simulink model "desulfuradora"  (Simulink 8.5)
settings: Solver=ode45  StartTime=0.0  StopTime=20000  RelTol=1e-3
undefined symbols (not defined in the file or in its folder): magnitude, Pump, SmartFuel, tabla, tank
settings Model: Creator=juanillo  LastModifiedBy=Jota
settings OptimizationCC: InitFltsAndDblsToZero=on
settings DebuggingCC: SaveWithParameterizedLinksMsg=none  SolverPrmCheckMsg=warning  FcnCallInpInsideContextMsg=UseLocalSettings
settings GRTTargetCC: TargetFcnLib=ansi_tfl_tmw.mat

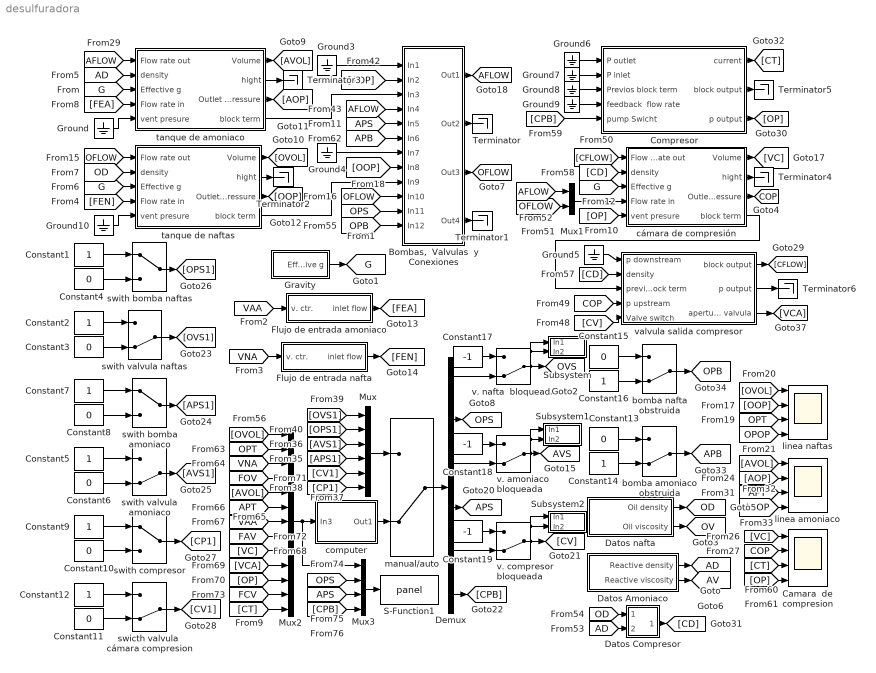
== system desulfuradora ==
  " bomba amoniaco obstruida" : ManualSwitch  CurrentSetting=0
  " bomba nafta obstruida" : ManualSwitch  CurrentSetting=0
  " linea amoniaco" : Scope  NumInputPorts=4
      settings: TickLabels=on  YMin=19~93100~36.9~210808  YMax=21~102900~37.1~232998  SaveName=tnafta2
  " linea naftas" : Scope  NumInputPorts=4
      settings: TickLabels=on  YMin=1~0~20~0  YMax=11~55000~110~200000  SaveName=tnafta
  " v. amoniaco  bloqueada" : ManualSwitch  CurrentSetting=0
  " v. compresor  bloqueada" : ManualSwitch  CurrentSetting=0
  " v. nafta  bloqueada" : ManualSwitch  CurrentSetting=0
  "Bombas,  Valvulas  y Conexiones" : Subsystem
  Camara  de compresion : Scope  NumInputPorts=4
      settings: TimeRange=2000  YMin=17.1501~1.45e+007~145~1.45e+007  YMax=18.9553~2.05e+007~162.5~2.05e+007  SaveName=camarac
  Compresor : Subsystem  AncestorBlock=SmartFuel/Pump  mask{V=350, P=2000, Rc=2, RO=0.2, L=20, Kb=0.35, Ki=0.5, J=2.5, A=2, R=250, E=0}
      mask prompts: V "Nominal Voltage"; P "Nominal Power"; Rc "rotor elec resistance"; RO "rotor mec. resitance"; L "rotor inductance"; Kb "Ind constant"; Ki "magres"; J "Rotor inertia"; A "valve section"; R "pump efficiency"; E "Last element (0/1)"
  Constant{1..2,5,7,9,12,14,16} (8 alike) : Constant
  Constant{3..4,6,8,10..11,13,15} (8 alike) : Constant  Value=0
  Constant17 : Constant  Value=-1
  Constant18 : Constant  Value=-1
  Constant19 : Constant  Value=-1
  Datos Amoniaco : Subsystem  AncestorBlock=SmartFuel/Fuel data  mask{ro=1000, mu=1.3}
      mask prompts: ro "Fuel density"; mu "Fuel viscosity"
  Datos Compresor : Subsystem
  Datos nafta : Subsystem  AncestorBlock=SmartFuel/Fuel data  mask{ro=1000, mu=1.3}
      mask prompts: ro "Fuel density"; mu "Fuel viscosity"
  Demux : Demux  Outputs=6
  Flujo de entrada amoniaco : Subsystem  mask{T=40, C=0.6}
      mask prompts: T "Inlet Period"; C "Flow"
  Flujo de entrada nafta : Subsystem  mask{T=40, C=0.4}
      mask prompts: T "Inlet period"; C "Flow"
  Gravity : Subsystem  AncestorBlock=SmartFuel/Aircraft data  mask{g=9.8, atitude=[0 0 0]}
      mask prompts: g "effective g"; atitude "Aircraft atitude"
  Ground{,3..10} (9 alike) : Ground
  Mux : Mux  Inputs=6
  Mux1 : Mux  Inputs=2
  Mux2 : Mux  Inputs=13
  Mux3 : Mux
  S-Function1 : S-Function  FunctionName=panel
  Subsystem : Subsystem
      mask Display: disp('FOV')
  Subsystem1 : Subsystem
      mask Display: disp('FAV')
  Subsystem2 : Subsystem
      mask Display: disp('FCV')
  Terminator{,1..6} (7 alike) : Terminator
  computer : Subsystem
      mask Display: disp('ordenador\n de control')
  cámara de compresión : Subsystem  AncestorBlock=SmartFuel/tank  mask{S=2, max=20, V0=0}
      mask prompts: S "Tank Geometrical Parameters"; max "Tank Max. Volume"; V0 "Initial Vol."
  manual/auto : ManualSwitch  CurrentSetting=0
  "swicth valvula  cámara compresion " : ManualSwitch  CurrentSetting=0
  swith bomba amoniaco : ManualSwitch
  swith bomba naftas : ManualSwitch
  swith compresor : ManualSwitch
  swith valvula amoniaco : ManualSwitch  CurrentSetting=0
  swith valvula naftas : ManualSwitch  CurrentSetting=0
  tanque de amoniaco : Subsystem  AncestorBlock=SmartFuel/tank  mask{S=2, max=20, V0=1}
      mask prompts: S "Tank Geometrical Parameters"; max "Tank Max. Volume"; V0 "Initial Vol."
  tanque de naftas : Subsystem  AncestorBlock=SmartFuel/tank  mask{S=2, max=20, V0=1}
      mask prompts: S "Tank Geometrical Parameters"; max "Tank Max. Volume"; V0 "Initial Vol."
  valvula salida compresor : Subsystem  mask{cv=0.5, T=0.1, A=0.2, E=1}
      mask prompts: cv "valve resistence"; T "aperture time"; A "Maximum valve aperture"; E "Last block (0/1)"
  tag scope: AD=global, AFLOW=global, APB=global, APS=global, AV=global, AVS=global, COP=global, G=global, OD=global, OFLOW=global, OPB=global, OPS=global, OV=global, OVS=global
  wires:
  Datos Amoniaco/1(Reactive density) -> [AD]
  Gravity/1(Effective g) -> [G]
  Datos Amoniaco/2(Reactive viscosity) -> [AV]
  Datos nafta/1(Oil density) -> [OD]
  Datos nafta/2(Oil viscosity) -> [OV]
  [AD] -> tanque de amoniaco/2(" density")
  [G] -> tanque de amoniaco/3(Effective g)
  [OD] -> tanque de naftas/2(" density")
  [G] -> tanque de naftas/3(Effective g)
  tanque de naftas/4(block term) -> "Bombas,  Valvulas  y Conexiones"/9(In9)
  cámara de compresión/3(Outlet Pressure) -> [COP]
  Mux1/1 -> cámara de compresión/4(Flow rate in)
  [G] -> cámara de compresión/3(Effective g)
  [OFLOW] -> tanque de naftas/1(Flow rate out)
  swith valvula naftas/1 -> [OVS1]
  Constant2/1 -> swith valvula naftas/1
  Constant3/1 -> swith valvula naftas/2
  cámara de compresión/1(Volume) -> [VC]
  tanque de amoniaco/1(Volume) -> [AVOL]
  tanque de naftas/1(Volume) -> [OVOL]
  tanque de amoniaco/3(Outlet Pressure) -> [AOP]
  tanque de naftas/3(Outlet Pressure) -> [OOP]
  [OPT] -> " linea naftas"/3
  [VC] -> Camara  de compresion/1
  [COP] -> Camara  de compresion/2
  [AFLOW] -> tanque de amoniaco/1(Flow rate out)
  [OVOL] -> " linea naftas"/1
  [OOP] -> " linea naftas"/2
  swith bomba naftas/1 -> [OPS1]
  Constant1/1 -> swith bomba naftas/1
  Constant4/1 -> swith bomba naftas/2
  swith valvula amoniaco/1 -> [AVS1]
  Constant5/1 -> swith valvula amoniaco/1
  Constant6/1 -> swith valvula amoniaco/2
  [APT] -> " linea amoniaco"/3
  [AVOL] -> " linea amoniaco"/1
  [AOP] -> " linea amoniaco"/2
  [APOP] -> " linea amoniaco"/4
  swith bomba amoniaco/1 -> [APS1]
  Constant7/1 -> swith bomba amoniaco/1
  Constant8/1 -> swith bomba amoniaco/2
  swith compresor/1 -> [CP1]
  Constant9/1 -> swith compresor/1
  Constant10/1 -> swith compresor/2
  Ground/1 -> tanque de amoniaco/5(vent presure)
  tanque de amoniaco/4(block term) -> "Bombas,  Valvulas  y Conexiones"/3(In3)
  Mux/1 -> manual/auto/1
  Demux/2 -> [OPS]
  Demux/3 -> " v. amoniaco  bloqueada"/2
  Demux/4 -> [APS]
  "swicth valvula  cámara compresion "/1 -> [CV1]
  Constant12/1 -> "swicth valvula  cámara compresion "/1
  Constant11/1 -> "swicth valvula  cámara compresion "/2
  Demux/6 -> [CPB]
  [OVS1] -> Mux/1
  [OPS1] -> Mux/2
  [AVS1] -> Mux/3
  [CV1] -> Mux/5
  [CP1] -> Mux/6
  [APS1] -> Mux/4
  tanque de naftas/2(hight) -> Terminator2/1
  tanque de amoniaco/2(hight) -> Terminator3/1
  valvula salida compresor/1(block output) -> [CFLOW]
  [CV] -> valvula salida compresor/5(Valve switch)
  Ground5/1 -> valvula salida compresor/1(p downstream)
  [COP] -> valvula salida compresor/4(p upstream)
  cámara de compresión/4(block term) -> valvula salida compresor/3(previous block term)
  cámara de compresión/2(hight) -> Terminator4/1
  Compresor/2(block output) -> Terminator5/1
  Compresor/3(p output) -> [OP]
  [OP] -> cámara de compresión/5(vent presure)
  [CFLOW] -> cámara de compresión/1(Flow rate out)
  [OFLOW] -> Mux1/2
  [AFLOW] -> Mux1/1
  Datos Compresor/1(Out3) -> [CD]
  [CD] -> cámara de compresión/2(" density")
  [CD] -> valvula salida compresor/2(" density")
  Ground6/1 -> Compresor/1(P outlet)
  Ground7/1 -> Compresor/2(P inlet)
  Ground8/1 -> Compresor/3(Previos block term)
  Ground9/1 -> Compresor/4(feedback  flow rate)
  [CPB] -> Compresor/5(pump Swicht)
  Compresor/1(current) -> [CT]
  [CT] -> Camara  de compresion/3
  [OP] -> Camara  de compresion/4
  Ground10/1 -> tanque de naftas/5(vent presure)
  " bomba amoniaco obstruida"/1 -> [APB]
  Constant13/1 -> " bomba amoniaco obstruida"/1
  Constant14/1 -> " bomba amoniaco obstruida"/2
  [AD] -> Datos Compresor/2(In2)
  [OD] -> Datos Compresor/1(In1)
  " bomba nafta obstruida"/1 -> [OPB]
  Constant15/1 -> " bomba nafta obstruida"/1
  Constant16/1 -> " bomba nafta obstruida"/2
  Mux2/1 -> Mux3/1, computer/1(In3)
  computer/1(Out1) -> manual/auto/2
  [OVOL] -> Mux2/1
  [OPT] -> Mux2/2
  " v. nafta  bloqueada"/1 -> Subsystem/2(In2), Subsystem/1(In1), [OVS]
  Demux/1 -> " v. nafta  bloqueada"/2
  Constant17/1 -> " v. nafta  bloqueada"/1
  " v. amoniaco  bloqueada"/1 -> [AVS], Subsystem1/2(In2), Subsystem1/1(In1)
  Constant18/1 -> " v. amoniaco  bloqueada"/1
  Demux/5 -> " v. compresor  bloqueada"/2
  " v. compresor  bloqueada"/1 -> [CV], Subsystem2/2(In2), Subsystem2/1(In1)
  [VNA] -> Mux2/3
  valvula salida compresor/3(apertura valvula) -> [VCA]
  valvula salida compresor/2(p output) -> Terminator6/1
  [AVOL] -> Mux2/5
  [APT] -> Mux2/6
  [VAA] -> Mux2/7
  [FOV] -> Mux2/4
  [VC] -> Mux2/9
  [VCA] -> Mux2/10
  [OP] -> Mux2/11
  [FAV] -> Mux2/8
  [FCV] -> Mux2/12
  [OPOP] -> " linea naftas"/4
  Mux3/1 -> S-Function1/1
  [OPS] -> Mux3/2
  [APS] -> Mux3/3
  [CPB] -> Mux3/4
  Constant19/1 -> " v. compresor  bloqueada"/1
  [APB] -> "Bombas,  Valvulas  y Conexiones"/6(In6)
  "Bombas,  Valvulas  y Conexiones"/2(Out2) -> Terminator/1
  Ground3/1 -> "Bombas,  Valvulas  y Conexiones"/1(In1)
  [AFLOW] -> "Bombas,  Valvulas  y Conexiones"/4(In4)
  [AOP] -> "Bombas,  Valvulas  y Conexiones"/2(In2)
  [APS] -> "Bombas,  Valvulas  y Conexiones"/5(In5)
  "Bombas,  Valvulas  y Conexiones"/1(Out1) -> [AFLOW]
  [OPB] -> "Bombas,  Valvulas  y Conexiones"/12(In12)
  "Bombas,  Valvulas  y Conexiones"/4(Out4) -> Terminator1/1
  Ground4/1 -> "Bombas,  Valvulas  y Conexiones"/7(In7)
  [OOP] -> "Bombas,  Valvulas  y Conexiones"/8(In8)
  [OFLOW] -> "Bombas,  Valvulas  y Conexiones"/10(In10)
  "Bombas,  Valvulas  y Conexiones"/3(Out3) -> [OFLOW]
  [OPS] -> "Bombas,  Valvulas  y Conexiones"/11(In11)
  manual/auto/1 -> Demux/1
  [VAA] -> Flujo de entrada amoniaco/1(v. ctr.)
  [VNA] -> Flujo de entrada nafta/1(v. ctr.)
  Flujo de entrada amoniaco/1(inlet flow) -> [FEA]
  Flujo de entrada nafta/1(inlet flow) -> [FEN]
  [FEN] -> tanque de naftas/4(Flow rate in)
  [FEA] -> tanque de amoniaco/4(Flow rate in)
  [CT] -> Mux2/13

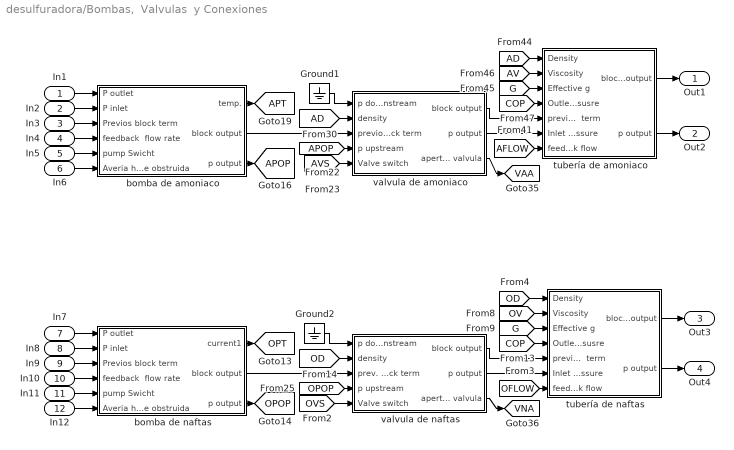
== system desulfuradora/Bombas,  Valvulas  y Conexiones ==
  In1 : Inport
  In2 : Inport  Port=2
  In3 : Inport  Port=3
  In4 : Inport  Port=4
  In5 : Inport  Port=5
  In6 : Inport  Port=6
  In7 : Inport  Port=7
  In8 : Inport  Port=8
  In9 : Inport  Port=9
  In10 : Inport  Port=10
  In11 : Inport  Port=11
  In12 : Inport  Port=12
  Ground1 : Ground
  Ground2 : Ground
  bomba de amoniaco : Subsystem  AncestorBlock=SmartFuel/Pump  mask{V=250, P=5000, Rc=2, RO=0.2, L=2, Kb=0.5, Ki=8, J=2.5, A=0.3, R=0.6, E=0}
      mask prompts: V "Nominal Voltage"; P "Nominal Power"; Rc "rotor elec resistance"; RO "rotor mec. resitance"; L "rotor inductance"; Kb "Ind constant"; Ki "magres"; J "Rotor inertia"; A "valve section"; R "pump efficiency"; E "Last element (0/1)"
  bomba de naftas : Subsystem  AncestorBlock=SmartFuel/Pump  mask{V=250, P=5000, Rc=2, RO=0.2, L=2, Kb=0.5, Ki=8, J=2.5, A=0.3, R=0.6, E=0}
      mask prompts: V "Nominal Voltage"; P "Nominal Power"; Rc "rotor elec resistance"; RO "rotor mec. resitance"; L "rotor inductance"; Kb "Ind constant"; Ki "magres"; J "Rotor inertia"; A "valve section"; R "pump efficiency"; E "Last element (0/1)"
  tubería de amoniaco : Subsystem  mask{PA=[0  0  0], D=0.3, L=2, R=0.00003, E=1}
      mask prompts: PA "Pipe atitude (Relative to landed aircraft)"; D "Pipe Diameter"; L "Pipe Length"; R "Pipe Rougness"; E "Last block (0/1)"
      mask init:
      | load re
      | load tabla
      | load eps_d
  tubería de naftas : Subsystem  mask{PA=[0  0  0], D=0.3, L=2, R=0.00003, E=1}
      mask prompts: PA "Pipe atitude (Relative to landed aircraft)"; D "Pipe Diameter"; L "Pipe Length"; R "Pipe Rougness"; E "Last block (0/1)"
      mask init:
      | load re
      | load tabla
      | load eps_d
  valvula de amoniaco : Subsystem  mask{cv=0.5, T=0.1, A=0.3, E=0}
      mask prompts: cv "valve resistence"; T "aperture time"; A "Maximum valve aperture"; E "Last block (0/1)"
  valvula de naftas : Subsystem  mask{cv=0.5, T=0.1, A=0.3, E=0}
      mask prompts: cv "valve resistence"; T "aperture time"; A "Maximum valve aperture"; E "Last block (0/1)"
  Out1 : Outport
  Out2 : Outport  Port=2
  Out3 : Outport  Port=3
  Out4 : Outport  Port=4
  tag scope: APOP=global, APT=global, OPOP=global, OPT=global, VAA=global, VNA=global
  wires:
  [AD] -> tubería de amoniaco/1(Density)
  valvula de amoniaco/3(apertura valvula) -> [VAA]
  valvula de amoniaco/1(block output) -> tubería de amoniaco/5(previous block  term)
  [COP] -> tubería de amoniaco/4(Outlet Presusre)
  [G] -> tubería de amoniaco/3(Effective g)
  [AV] -> tubería de amoniaco/2(Viscosity)
  [AFLOW] -> tubería de amoniaco/7(feedbak flow)
  valvula de amoniaco/2(p output) -> tubería de amoniaco/6(Inlet Pressure)
  Ground1/1 -> valvula de amoniaco/1(p downstream)
  [AVS] -> valvula de amoniaco/5(Valve switch)
  [APOP] -> valvula de amoniaco/4(p upstream)
  [AD] -> valvula de amoniaco/2(" density")
  bomba de amoniaco/2(block output) -> valvula de amoniaco/3(previous block term)
  bomba de amoniaco/3(p output) -> [APOP]
  bomba de amoniaco/1(temp.) -> [APT]
  [OD] -> tubería de naftas/1(Density)
  valvula de naftas/3(apertura valvula) -> [VNA]
  Ground2/1 -> valvula de naftas/1(p downstream)
  [OPOP] -> valvula de naftas/4(p upstream)
  bomba de naftas/3(p output) -> [OPOP]
  bomba de naftas/1(current1) -> [OPT]
  [OD] -> valvula de naftas/2(" density")
  [COP] -> tubería de naftas/4(Outlet Presusre)
  [OFLOW] -> tubería de naftas/7(feedbak flow)
  [G] -> tubería de naftas/3(Effective g)
  [OV] -> tubería de naftas/2(Viscosity)
  valvula de naftas/1(block output) -> tubería de naftas/5(previous block  term)
  valvula de naftas/2(p output) -> tubería de naftas/6(Inlet Pressure)
  bomba de naftas/2(block output) -> valvula de naftas/3(prev. block term)
  [OVS] -> valvula de naftas/5(Valve switch)
  tubería de amoniaco/1(block output) -> Out1/1
  In1/1 -> bomba de amoniaco/1(P outlet)
  In2/1 -> bomba de amoniaco/2(P inlet)
  In3/1 -> bomba de amoniaco/3(Previos block term)
  tubería de amoniaco/2(p output) -> Out2/1
  In4/1 -> bomba de amoniaco/4(feedback  flow rate)
  In5/1 -> bomba de amoniaco/5(pump Swicht)
  In6/1 -> bomba de amoniaco/6(Averia helice obstruida)
  tubería de naftas/1(block output) -> Out3/1
  In7/1 -> bomba de naftas/1(P outlet)
  In8/1 -> bomba de naftas/2(P inlet)
  In9/1 -> bomba de naftas/3(Previos block term)
  tubería de naftas/2(p output) -> Out4/1
  In10/1 -> bomba de naftas/4(feedback  flow rate)
  In11/1 -> bomba de naftas/5(pump Swicht)
  In12/1 -> bomba de naftas/6(Averia helice obstruida)

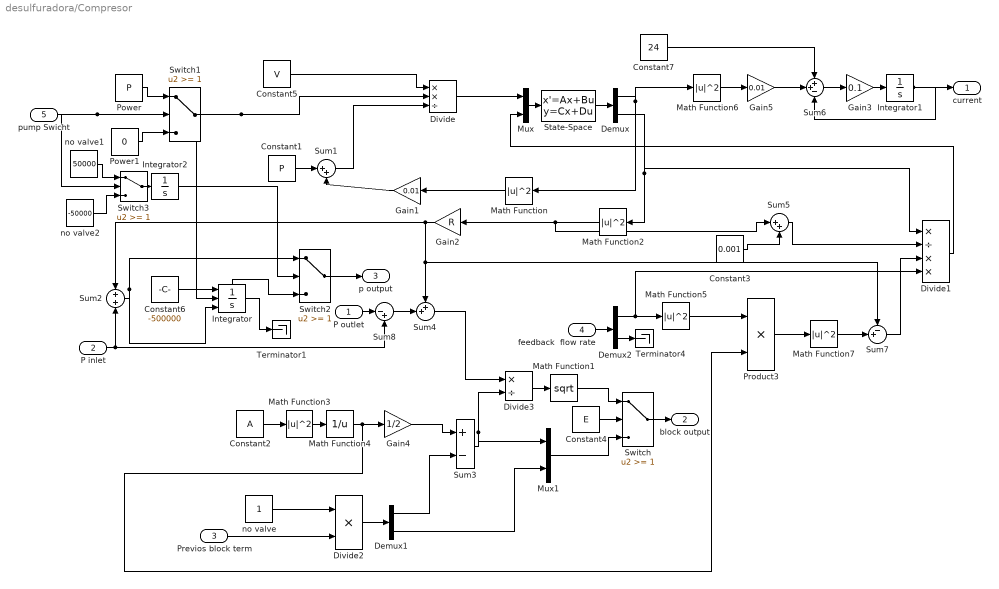
== system desulfuradora/Compresor ==
  P outlet : Inport
  P inlet : Inport  Port=2
  Previos block term : Inport  Port=3
  feedback  flow rate : Inport  Port=4
  pump Swicht : Inport  Port=5
  Constant1 : Constant  Value=P
  Constant2 : Constant  Value=A
  Constant3 : Constant  Value=0.001
  Constant4 : Constant  Value=E
  Constant5 : Constant  Value=V
  Constant6 : Constant  Value=-500000
  Constant7 : Constant  Value=24
  Demux : Demux  Outputs=2
  Demux1 : Demux  Outputs=2
  Demux2 : Demux  Outputs=2
  Divide : Product  Inputs=**/
  Divide1 : Product  Inputs=*/**
  Divide2 : Product  Inputs=**
  Divide3 : Product  Inputs=*/
  Gain1 : Gain  Gain=0.01
  Gain2 : Gain  Gain=R
  Gain3 : Gain  Gain=0.1
  Gain4 : Gain  Gain=1/2
  Gain5 : Gain  Gain=0.01
  Integrator : Integrator  ExternalReset=falling  InitialConditionSource=external  LimitOutput=on  LowerSaturationLimit=0  ShowStatePort=on
  Integrator1 : Integrator  InitialCondition=24
  Integrator2 : Integrator  LimitOutput=on  UpperSaturationLimit=1  LowerSaturationLimit=0
  Math Function{,2..3,5..7} (6 alike) : Math  Operator=magnitude^2  SaturateOnIntegerOverflow=on
  Math Function1 : Math  Operator=sqrt  SaturateOnIntegerOverflow=on
  Math Function4 : Math  Operator=reciprocal  SaturateOnIntegerOverflow=on
  Mux : Mux  Inputs=2
  Mux1 : Mux  Inputs=2
  Power : Constant  Value=P
  Power1 : Constant  Value=0
  Product3 : Product  RndMeth=Zero
  State-Space : StateSpace  A=[-Rc/L -Kb/L;Ki/J -RO/J]  B=[1/L 0;0 -1/J]  C=[1 0;0 1]  D=[0 0;0 0]  X0=0
  Sum1 : Sum  Inputs=|++
  Sum2 : Sum
  Sum3 : Sum  Inputs=+-
  Sum4 : Sum  Inputs=++|
  Sum5 : Sum  Inputs=|++
  Sum6 : Sum  Inputs=++-
  Sum7 : Sum  Inputs=-+|
  Sum8 : Sum  Inputs=|-+
  Switch{,1..3} (4 alike) : Switch  Threshold=1
  Terminator1 : Terminator
  Terminator4 : Terminator
  no valve : Constant
  no valve1 : Constant  Value=50000
  no valve2 : Constant  Value=-50000
  current : Outport
  block output : Outport  Port=2
  p output : Outport  Port=3
  wires:
  Mux/1 -> State-Space/1
  P outlet/1 -> Sum8/1
  State-Space/1 -> Demux/1
  Demux/1 -> Math Function/1, Math Function6/1
  Constant1/1 -> Sum1/1
  Demux/2 -> Divide1/1, Math Function2/1
  Math Function2/1 -> Gain2/1, Sum5/1
  P inlet/1 -> Sum2/2, Sum8/2
  Math Function3/1 -> Math Function4/1
  Math Function4/1 -> Gain4/1, Product3/2
  Constant2/1 -> Math Function3/1
  Divide2/1 -> Demux1/1
  no valve/1 -> Divide2/1
  Previos block term/1 -> Divide2/2
  Sum2/1 -> Switch2/1, Integrator/3
  Divide3/1 -> Math Function1/1
  Gain4/1 -> Sum3/1
  Sum3/1 -> Divide3/2, Mux1/1
  Constant4/1 -> Switch/2
  Switch/1 -> block output/1
  Mux1/1 -> Switch/3
  Math Function1/1 -> Switch/1
  Demux1/2 -> Mux1/2
  Power/1 -> Switch1/1
  Power1/1 -> Switch1/3
  pump Swicht/1 -> Switch1/2, Switch3/2
  feedback  flow rate/1 -> Demux2/1
  Demux2/2 -> Terminator4/1
  Demux1/1 -> Sum3/2
  Sum8/1 -> Sum4/2
  Sum4/1 -> Divide3/1
  Gain2/1 -> Sum2/1, Sum4/1, Sum7/1
  Demux2/1 -> Math Function5/1, Divide1/4
  Sum1/1 -> Divide/3
  Switch1/1 -> Divide/2, Integrator/2
  Constant5/1 -> Divide/1
  Gain1/1 -> Sum1/2
  Math Function/1 -> Gain1/1
  Divide/1 -> Mux/1
  Math Function5/1 -> Product3/1
  Product3/1 -> Math Function7/1
  Constant3/1 -> Sum5/2
  Math Function7/1 -> Sum7/2
  Sum7/1 -> Divide1/3
  Sum5/1 -> Divide1/2
  Divide1/1 -> Mux/2
  Constant6/1 -> Integrator/1
  Switch2/1 -> p output/1
  Integrator1/1 -> Sum6/3, current/1
  Constant7/1 -> Sum6/1
  Sum6/1 -> Gain3/1
  Gain3/1 -> Integrator1/1
  Gain5/1 -> Sum6/2
  Math Function6/1 -> Gain5/1
  Integrator/State -> Switch2/3
  Integrator/1 -> Terminator1/1
  Switch3/1 -> Integrator2/1
  no valve1/1 -> Switch3/1
  no valve2/1 -> Switch3/3
  Integrator2/1 -> Switch2/2

== system desulfuradora/Datos Amoniaco ==
  FD : Constant  Value=ro
  FV : Constant  Value=mu
  Reactive density : Outport
  Reactive viscosity : Outport  Port=2
  wires:
  FV/1 -> Reactive viscosity/1
  FD/1 -> Reactive density/1

== system desulfuradora/Datos Compresor ==
  In1 : Inport
  In2 : Inport  Port=2
  Gain3 : Gain  Gain=1/2
  Sum1 : Sum
  Out3 : Outport
  wires:
  In2/1 -> Sum1/2
  In1/1 -> Sum1/1
  Gain3/1 -> Out3/1
  Sum1/1 -> Gain3/1

== system desulfuradora/Datos nafta ==
  FD : Constant  Value=ro
  FV : Constant  Value=mu
  Oil density : Outport
  Oil viscosity : Outport  Port=2
  wires:
  FV/1 -> Oil viscosity/1
  FD/1 -> Oil density/1

== system desulfuradora/Flujo de entrada amoniaco ==
  v. ctr. : Inport
  Constant20 : Constant  Value=0
  Pulse Generator : DiscretePulseGenerator  PulseType=Time based  Amplitude=C  Period=T  PulseWidth=50
  Switch : Switch  Criteria=u2 > Threshold  Threshold=-1
  inlet flow : Outport
  wires:
  Pulse Generator/1 -> Switch/3
  Constant20/1 -> Switch/1
  v. ctr./1 -> Switch/2
  Switch/1 -> inlet flow/1

== system desulfuradora/Flujo de entrada nafta ==
  v. ctr. : Inport
  Constant20 : Constant  Value=0
  Pulse Generator : DiscretePulseGenerator  PulseType=Time based  Amplitude=C  Period=T  PulseWidth=50
  Switch : Switch  Criteria=u2 > Threshold  Threshold=-1
  inlet flow : Outport
  wires:
  Pulse Generator/1 -> Switch/3
  Constant20/1 -> Switch/1
  v. ctr./1 -> Switch/2
  Switch/1 -> inlet flow/1

== system desulfuradora/Gravity ==
  EG : Constant  Value=g
  Effective g : Outport
  wires:
  EG/1 -> Effective g/1

== system desulfuradora/Subsystem ==
  In1 : Inport
  In2 : Inport  Port=2
  Constant20 : Constant
  Integrator : Integrator  LimitOutput=on  UpperSaturationLimit=1  LowerSaturationLimit=-1
  Switch : Switch
  tag scope: FOV=global
  wires:
  Switch/1 -> Integrator/1
  Constant20/1 -> Switch/1
  Integrator/1 -> [FOV]
  In1/1 -> Switch/2
  In2/1 -> Switch/3

== system desulfuradora/Subsystem1 ==
  In1 : Inport
  In2 : Inport  Port=2
  Constant20 : Constant
  Integrator : Integrator  LimitOutput=on  UpperSaturationLimit=1  LowerSaturationLimit=-1
  Switch : Switch
  tag scope: FAV=global
  wires:
  Switch/1 -> Integrator/1
  Constant20/1 -> Switch/1
  Integrator/1 -> [FAV]
  In1/1 -> Switch/2
  In2/1 -> Switch/3

== system desulfuradora/Subsystem2 ==
  In1 : Inport
  In2 : Inport  Port=2
  Constant20 : Constant
  Integrator : Integrator  LimitOutput=on  UpperSaturationLimit=1  LowerSaturationLimit=-1
  Switch : Switch
  tag scope: FCV=global
  wires:
  Switch/1 -> Integrator/1
  Constant20/1 -> Switch/1
  Integrator/1 -> [FCV]
  In1/1 -> Switch/2
  In2/1 -> Switch/3

== system desulfuradora/computer ==
  In3 : Inport
  Data Store Memory : DataStoreMemory  InitialValue=[-1, -1, -1, -1, -1, -1, -1, -1, -1, -1, -1, -1]
  Data Store Read : DataStoreRead  SampleTime=0
  Data Store Write : DataStoreWrite
  Demux : Demux  Outputs=2
  Mux : Mux  Inputs=2
  S-Function : S-Function  FunctionName=controlador
  Out1 : Outport
  wires:
  S-Function/1 -> Demux/1
  Demux/2 -> Data Store Write/1
  Demux/1 -> Out1/1
  Mux/1 -> S-Function/1
  In3/1 -> Mux/1
  Data Store Read/1 -> Mux/2

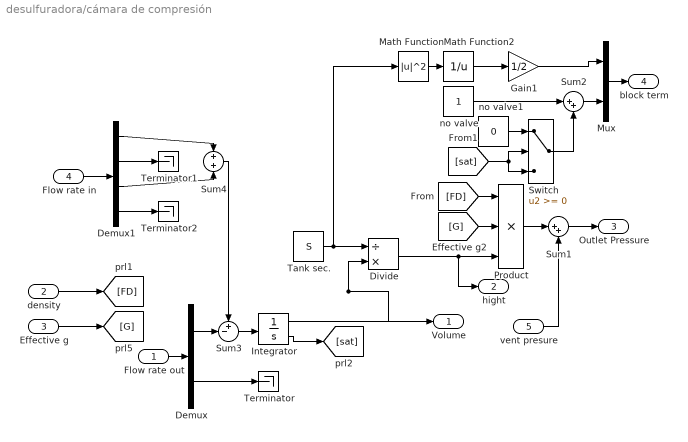
== system desulfuradora/cámara de compresión ==
  Flow rate out : Inport
  " density" : Inport  Port=2
  Effective g : Inport  Port=3
  Flow rate in : Inport  Port=4
  vent presure : Inport  Port=5
  Demux : Demux  Outputs=2
  Demux1 : Demux
  Divide : Product  Inputs=/*
  Gain1 : Gain  Gain=1/2
  Integrator : Integrator  InitialCondition=V0  LimitOutput=on  UpperSaturationLimit=max  LowerSaturationLimit=0  ShowSaturationPort=on
  Math Function1 : Math  Operator=magnitude^2  SaturateOnIntegerOverflow=on
  Math Function2 : Math  Operator=reciprocal  SaturateOnIntegerOverflow=on
  Mux : Mux  Inputs=2
  Product : Product  Inputs=3  RndMeth=Zero
  Sum1 : Sum  Inputs=|++
  Sum2 : Sum  Inputs=|++
  Sum3 : Sum  Inputs=+-|
  Sum4 : Sum
  Switch : Switch
  Tank sec. : Constant  Value=S
  Terminator : Terminator
  Terminator1 : Terminator
  Terminator2 : Terminator
  no valve : Constant
  no valve1 : Constant  Value=0
  Volume : Outport
  hight : Outport  Port=2
  Outlet Pressure : Outport  Port=3
  block term : Outport  Port=4
  wires:
  vent presure/1 -> Sum1/2
  Product/1 -> Sum1/1
  Sum1/1 -> Outlet Pressure/1
  Gain1/1 -> Mux/1
  Mux/1 -> block term/1
  Math Function2/1 -> Gain1/1
  Math Function1/1 -> Math Function2/1
  Tank sec./1 -> Math Function1/1, Divide/1
  [G] -> Product/2
  [FD] -> Product/1
  Effective g/1 -> [G]
  " density"/1 -> [FD]
  Divide/1 -> Product/3, hight/1
  Sum2/1 -> Mux/2
  no valve/1 -> Sum2/1
  Integrator/2 -> [sat]
  [sat] -> Switch/2, Switch/3
  no valve1/1 -> Switch/1
  Switch/1 -> Sum2/2
  Flow rate out/1 -> Demux/1
  Demux/2 -> Terminator/1
  Integrator/1 -> Divide/2, Volume/1
  Demux/1 -> Sum3/2
  Sum3/1 -> Integrator/1
  Flow rate in/1 -> Demux1/1
  Demux1/2 -> Terminator1/1
  Demux1/4 -> Terminator2/1
  Demux1/1 -> Sum4/1
  Demux1/3 -> Sum4/2
  Sum4/1 -> Sum3/1

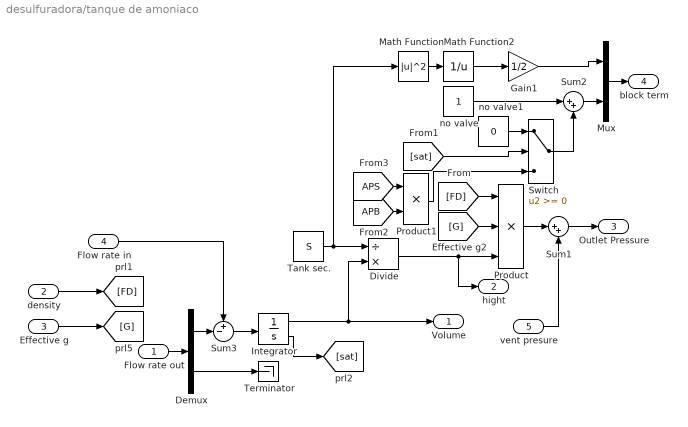
== system desulfuradora/tanque de amoniaco ==
  Flow rate out : Inport
  " density" : Inport  Port=2
  Effective g : Inport  Port=3
  Flow rate in : Inport  Port=4
  vent presure : Inport  Port=5
  Demux : Demux  Outputs=2
  Divide : Product  Inputs=/*
  Gain1 : Gain  Gain=1/2
  Integrator : Integrator  InitialCondition=V0  LimitOutput=on  UpperSaturationLimit=max  LowerSaturationLimit=0  ShowSaturationPort=on
  Math Function1 : Math  Operator=magnitude^2  SaturateOnIntegerOverflow=on
  Math Function2 : Math  Operator=reciprocal  SaturateOnIntegerOverflow=on
  Mux : Mux  Inputs=2
  Product : Product  Inputs=3  RndMeth=Zero
  Product1 : Product  RndMeth=Zero
  Sum1 : Sum  Inputs=|++
  Sum2 : Sum  Inputs=|++
  Sum3 : Sum  Inputs=+-|
  Switch : Switch
  Tank sec. : Constant  Value=S
  Terminator : Terminator
  no valve : Constant
  no valve1 : Constant  Value=0
  Volume : Outport
  hight : Outport  Port=2
  Outlet Pressure : Outport  Port=3
  block term : Outport  Port=4
  wires:
  vent presure/1 -> Sum1/2
  Product/1 -> Sum1/1
  Sum1/1 -> Outlet Pressure/1
  Gain1/1 -> Mux/1
  Mux/1 -> block term/1
  Math Function2/1 -> Gain1/1
  Math Function1/1 -> Math Function2/1
  Tank sec./1 -> Math Function1/1, Divide/1
  [G] -> Product/2
  [FD] -> Product/1
  Effective g/1 -> [G]
  " density"/1 -> [FD]
  Divide/1 -> Product/3, hight/1
  Sum2/1 -> Mux/2
  no valve/1 -> Sum2/1
  Integrator/2 -> [sat]
  [sat] -> Switch/2
  no valve1/1 -> Switch/1
  Switch/1 -> Sum2/2
  Flow rate in/1 -> Sum3/1
  Flow rate out/1 -> Demux/1
  Demux/2 -> Terminator/1
  Integrator/1 -> Divide/2, Volume/1
  Demux/1 -> Sum3/2
  Sum3/1 -> Integrator/1
  Product1/1 -> Switch/3
  [APS] -> Product1/1
  [APB] -> Product1/2

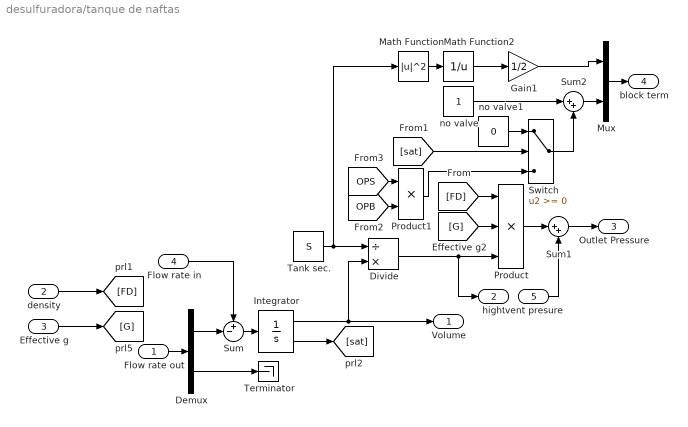
== system desulfuradora/tanque de naftas ==
  Flow rate out : Inport
  " density" : Inport  Port=2
  Effective g : Inport  Port=3
  Flow rate in : Inport  Port=4
  vent presure : Inport  Port=5
  Demux : Demux  Outputs=2
  Divide : Product  Inputs=/*
  Gain1 : Gain  Gain=1/2
  Integrator : Integrator  InitialCondition=V0  LimitOutput=on  UpperSaturationLimit=max  LowerSaturationLimit=0  ShowSaturationPort=on
  Math Function1 : Math  Operator=magnitude^2  SaturateOnIntegerOverflow=on
  Math Function2 : Math  Operator=reciprocal  SaturateOnIntegerOverflow=on
  Mux : Mux  Inputs=2
  Product : Product  Inputs=3  RndMeth=Zero
  Product1 : Product  RndMeth=Zero
  Sum : Sum  Inputs=+-|
  Sum1 : Sum  Inputs=|++
  Sum2 : Sum  Inputs=|++
  Switch : Switch
  Tank sec. : Constant  Value=S
  Terminator : Terminator
  no valve : Constant
  no valve1 : Constant  Value=0
  Volume : Outport
  hight : Outport  Port=2
  Outlet Pressure : Outport  Port=3
  block term : Outport  Port=4
  wires:
  Product/1 -> Sum1/1
  Sum1/1 -> Outlet Pressure/1
  Gain1/1 -> Mux/1
  Mux/1 -> block term/1
  Math Function2/1 -> Gain1/1
  Math Function1/1 -> Math Function2/1
  Tank sec./1 -> Math Function1/1, Divide/1
  [G] -> Product/2
  [FD] -> Product/1
  Effective g/1 -> [G]
  " density"/1 -> [FD]
  Divide/1 -> Product/3, hight/1
  Sum2/1 -> Mux/2
  no valve/1 -> Sum2/1
  Integrator/2 -> [sat]
  [sat] -> Switch/2
  no valve1/1 -> Switch/1
  Switch/1 -> Sum2/2
  Flow rate in/1 -> Sum/1
  Flow rate out/1 -> Demux/1
  Demux/2 -> Terminator/1
  Integrator/1 -> Divide/2, Volume/1
  Demux/1 -> Sum/2
  Sum/1 -> Integrator/1
  vent presure/1 -> Sum1/2
  Product1/1 -> Switch/3
  [OPS] -> Product1/1
  [OPB] -> Product1/2

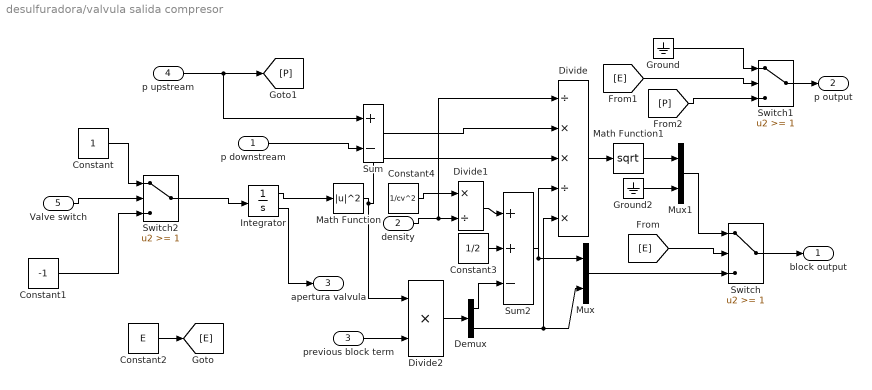
== system desulfuradora/valvula salida compresor ==
  p downstream : Inport
  " density" : Inport  Port=2
  previous block term : Inport  Port=3
  p upstream : Inport  Port=4
  Valve switch : Inport  Port=5
  Constant : Constant
  Constant1 : Constant  Value=-1
  Constant2 : Constant  Value=E
  Constant3 : Constant  Value=1/2
  Constant4 : Constant  Value=1/cv^2
  Demux : Demux  Outputs=2
  Divide : Product  Inputs=/**/*
  Divide1 : Product  Inputs=*/
  Divide2 : Product  Inputs=**
  Ground : Ground
  Ground2 : Ground
  Integrator : Integrator  LimitOutput=on  UpperSaturationLimit=A  LowerSaturationLimit=0  ShowSaturationPort=on
  Math Function : Math  Operator=magnitude^2  SaturateOnIntegerOverflow=on
  Math Function1 : Math  Operator=sqrt  SaturateOnIntegerOverflow=on
  Mux : Mux  Inputs=2
  Mux1 : Mux  Inputs=2
  Sum : Sum  Inputs=+-
  Sum2 : Sum  Inputs=++-
  Switch : Switch  Threshold=1
  Switch1 : Switch  Threshold=1
  Switch2 : Switch  Threshold=1
  block output : Outport
  p output : Outport  Port=2
  apertura valvula : Outport  Port=3
  wires:
  Constant3/1 -> Sum2/2
  Sum2/1 -> Mux/1, Divide/4
  Math Function/1 -> Divide2/1, Divide/3
  Divide1/1 -> Sum2/1
  Constant4/1 -> Divide1/1
  " density"/1 -> Divide1/2, Divide/1
  Switch1/1 -> p output/1
  Constant2/1 -> [E]
  [E] -> Switch1/2
  Ground/1 -> Switch1/1
  p upstream/1 -> [P], Sum/1
  [P] -> Switch1/3
  Constant/1 -> Switch2/1
  Switch2/1 -> Integrator/1
  Constant1/1 -> Switch2/3
  Valve switch/1 -> Switch2/2
  p downstream/1 -> Sum/2
  [E] -> Switch/2
  previous block term/1 -> Divide2/2
  Divide2/1 -> Demux/1
  Demux/1 -> Sum2/3
  Demux/2 -> Mux/2, Divide/5
  Switch/1 -> block output/1
  Mux/1 -> Switch/3
  Sum/1 -> Divide/2
  Divide/1 -> Math Function1/1
  Integrator/1 -> Math Function/1
  Math Function1/1 -> Mux1/1
  Ground2/1 -> Mux1/2
  Mux1/1 -> Switch/1
  Integrator/2 -> apertura valvula/1

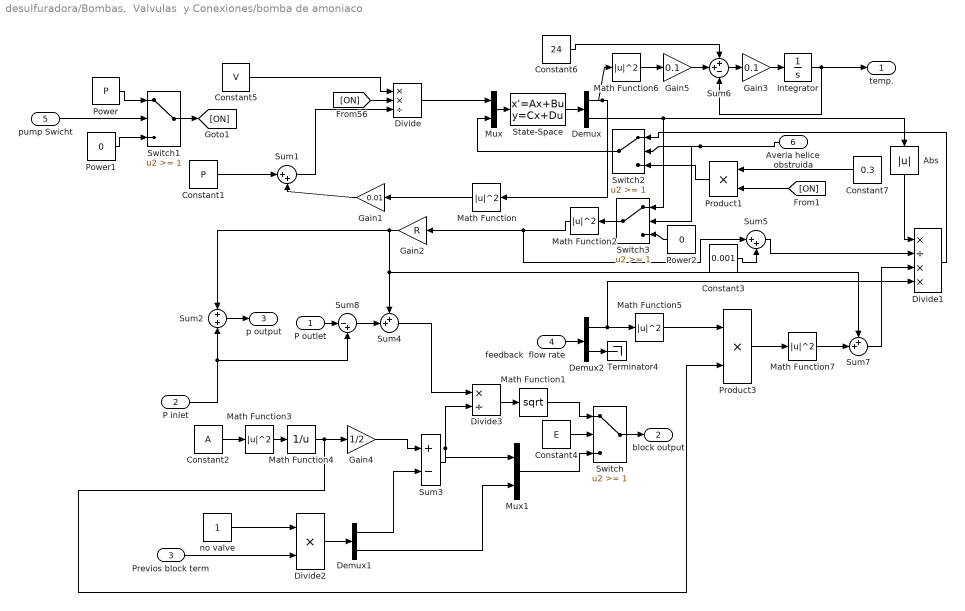
== system desulfuradora/Bombas,  Valvulas  y Conexiones/bomba de amoniaco ==
  P outlet : Inport
  P inlet : Inport  Port=2
  Previos block term : Inport  Port=3
  feedback  flow rate : Inport  Port=4
  pump Swicht : Inport  Port=5
  Averia helice obstruida : Inport  Port=6
  Abs : Abs
  Constant1 : Constant  Value=P
  Constant2 : Constant  Value=A
  Constant3 : Constant  Value=0.001
  Constant4 : Constant  Value=E
  Constant5 : Constant  Value=V
  Constant6 : Constant  Value=24
  Constant7 : Constant  Value=0.3
  Demux : Demux  Outputs=2
  Demux1 : Demux  Outputs=2
  Demux2 : Demux  Outputs=2
  Divide : Product  Inputs=**/
  Divide1 : Product  Inputs=*/**
  Divide2 : Product  Inputs=**
  Divide3 : Product  Inputs=*/
  Gain1 : Gain  Gain=0.01
  Gain2 : Gain  Gain=R
  Gain3 : Gain  Gain=0.1
  Gain4 : Gain  Gain=1/2
  Gain5 : Gain  Gain=0.1
  Integrator : Integrator  InitialCondition=24
  Math Function{,2..3,5..7} (6 alike) : Math  Operator=magnitude^2  SaturateOnIntegerOverflow=on
  Math Function1 : Math  Operator=sqrt  SaturateOnIntegerOverflow=on
  Math Function4 : Math  Operator=reciprocal  SaturateOnIntegerOverflow=on
  Mux : Mux  Inputs=2
  Mux1 : Mux  Inputs=2
  Power : Constant  Value=P
  Power1 : Constant  Value=0
  Power2 : Constant  Value=0
  Product1 : Product  RndMeth=Zero
  Product3 : Product  RndMeth=Zero
  State-Space : StateSpace  A=[-Rc/L -Kb/L;Ki/J -RO/J]  B=[1/L 0;0 -1/J]  C=[1 0;0 1]  D=[0 0;0 0]  X0=0
  Sum1 : Sum  Inputs=|++
  Sum2 : Sum
  Sum3 : Sum  Inputs=+-
  Sum4 : Sum  Inputs=++|
  Sum5 : Sum  Inputs=|++
  Sum6 : Sum  Inputs=++-
  Sum7 : Sum  Inputs=++|
  Sum8 : Sum  Inputs=|-+
  Switch{,1..3} (4 alike) : Switch  Threshold=1
  Terminator4 : Terminator
  no valve : Constant
  temp. : Outport
  block output : Outport  Port=2
  p output : Outport  Port=3
  wires:
  Mux/1 -> State-Space/1
  P outlet/1 -> Sum8/1
  State-Space/1 -> Demux/1
  Demux/1 -> Math Function/1, Math Function6/1
  Constant1/1 -> Sum1/1
  Math Function2/1 -> Gain2/1, Sum5/1
  P inlet/1 -> Sum2/2, Sum8/2
  Math Function3/1 -> Math Function4/1
  Math Function4/1 -> Gain4/1, Product3/2
  Constant2/1 -> Math Function3/1
  Divide2/1 -> Demux1/1
  no valve/1 -> Divide2/1
  Previos block term/1 -> Divide2/2
  Sum2/1 -> p output/1
  Divide3/1 -> Math Function1/1
  Gain4/1 -> Sum3/1
  Sum3/1 -> Divide3/2, Mux1/1
  Constant4/1 -> Switch/2
  Switch/1 -> block output/1
  Mux1/1 -> Switch/3
  Math Function1/1 -> Switch/1
  Demux1/2 -> Mux1/2
  Power/1 -> Switch1/1
  Power1/1 -> Switch1/3
  pump Swicht/1 -> Switch1/2
  feedback  flow rate/1 -> Demux2/1
  Demux2/2 -> Terminator4/1
  Demux1/1 -> Sum3/2
  Sum8/1 -> Sum4/2
  Sum4/1 -> Divide3/1
  Gain2/1 -> Sum2/1, Sum4/1, Sum7/1
  Demux2/1 -> Math Function5/1, Divide1/4
  Sum1/1 -> Divide/3
  Constant5/1 -> Divide/1
  Gain1/1 -> Sum1/2
  Math Function/1 -> Gain1/1
  Divide/1 -> Mux/1
  Math Function5/1 -> Product3/1
  Product3/1 -> Math Function7/1
  Constant3/1 -> Sum5/2
  Math Function7/1 -> Sum7/2
  Sum7/1 -> Divide1/3
  Sum5/1 -> Divide1/2
  Integrator/1 -> temp./1, Sum6/3
  Constant6/1 -> Sum6/1
  Divide1/1 -> Switch2/1
  Averia helice obstruida/1 -> Switch2/2, Switch3/2
  Switch2/1 -> Mux/2
  Switch1/1 -> [ON]
  [ON] -> Divide/2
  [ON] -> Product1/2
  Product1/1 -> Switch2/3
  Constant7/1 -> Product1/1
  Demux/2 -> Switch3/1, Abs/1
  Switch3/1 -> Math Function2/1
  Power2/1 -> Switch3/3
  Abs/1 -> Divide1/1
  Gain3/1 -> Integrator/1
  Sum6/1 -> Gain3/1
  Gain5/1 -> Sum6/2
  Math Function6/1 -> Gain5/1

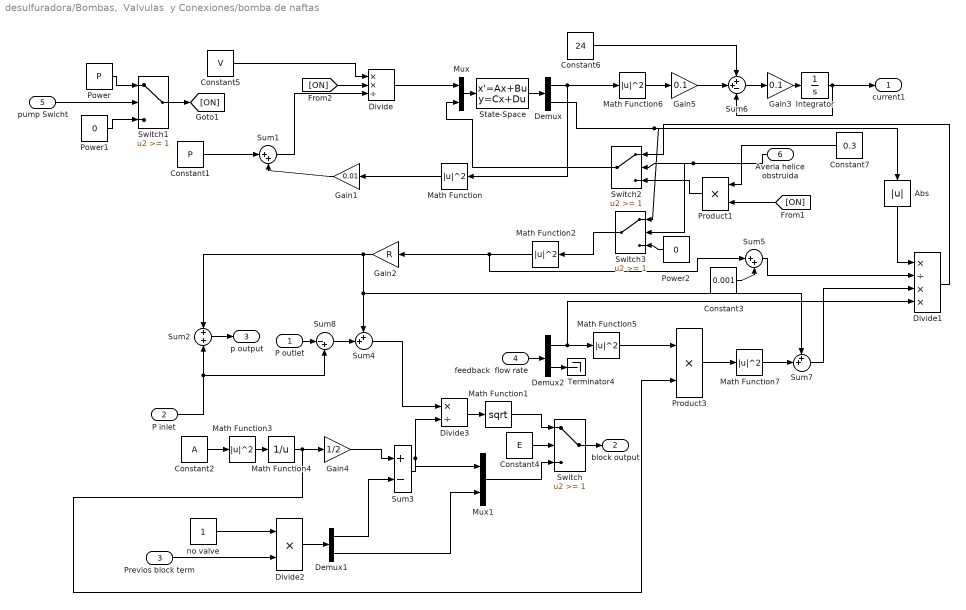
== system desulfuradora/Bombas,  Valvulas  y Conexiones/bomba de naftas ==
  P outlet : Inport
  P inlet : Inport  Port=2
  Previos block term : Inport  Port=3
  feedback  flow rate : Inport  Port=4
  pump Swicht : Inport  Port=5
  Averia helice obstruida : Inport  Port=6
  Abs : Abs
  Constant1 : Constant  Value=P
  Constant2 : Constant  Value=A
  Constant3 : Constant  Value=0.001
  Constant4 : Constant  Value=E
  Constant5 : Constant  Value=V
  Constant6 : Constant  Value=24
  Constant7 : Constant  Value=0.3
  Demux : Demux  Outputs=2
  Demux1 : Demux  Outputs=2
  Demux2 : Demux  Outputs=2
  Divide : Product  Inputs=**/
  Divide1 : Product  Inputs=*/**
  Divide2 : Product  Inputs=**
  Divide3 : Product  Inputs=*/
  Gain1 : Gain  Gain=0.01
  Gain2 : Gain  Gain=R
  Gain3 : Gain  Gain=0.1
  Gain4 : Gain  Gain=1/2
  Gain5 : Gain  Gain=0.1
  Integrator : Integrator  InitialCondition=24
  Math Function{,2..3,5..7} (6 alike) : Math  Operator=magnitude^2  SaturateOnIntegerOverflow=on
  Math Function1 : Math  Operator=sqrt  SaturateOnIntegerOverflow=on
  Math Function4 : Math  Operator=reciprocal  SaturateOnIntegerOverflow=on
  Mux : Mux  Inputs=2
  Mux1 : Mux  Inputs=2
  Power : Constant  Value=P
  Power1 : Constant  Value=0
  Power2 : Constant  Value=0
  Product1 : Product  RndMeth=Zero
  Product3 : Product  RndMeth=Zero
  State-Space : StateSpace  A=[-Rc/L -Kb/L;Ki/J -RO/J]  B=[1/L 0;0 -1/J]  C=[1 0;0 1]  D=[0 0;0 0]  X0=0
  Sum1 : Sum  Inputs=|++
  Sum2 : Sum
  Sum3 : Sum  Inputs=+-
  Sum4 : Sum  Inputs=++|
  Sum5 : Sum  Inputs=|++
  Sum6 : Sum  Inputs=++-
  Sum7 : Sum  Inputs=++|
  Sum8 : Sum  Inputs=|-+
  Switch{,1..3} (4 alike) : Switch  Threshold=1
  Terminator4 : Terminator
  no valve : Constant
  current1 : Outport
  block output : Outport  Port=2
  p output : Outport  Port=3
  wires:
  Mux/1 -> State-Space/1
  P outlet/1 -> Sum8/1
  State-Space/1 -> Demux/1
  Demux/1 -> Math Function/1, Math Function6/1
  Constant1/1 -> Sum1/1
  Demux/2 -> Switch3/1, Abs/1
  Math Function2/1 -> Gain2/1, Sum5/1
  P inlet/1 -> Sum2/2, Sum8/2
  Math Function3/1 -> Math Function4/1
  Math Function4/1 -> Gain4/1, Product3/2
  Constant2/1 -> Math Function3/1
  Divide2/1 -> Demux1/1
  no valve/1 -> Divide2/1
  Previos block term/1 -> Divide2/2
  Sum2/1 -> p output/1
  Divide3/1 -> Math Function1/1
  Gain4/1 -> Sum3/1
  Sum3/1 -> Divide3/2, Mux1/1
  Constant4/1 -> Switch/2
  Switch/1 -> block output/1
  Mux1/1 -> Switch/3
  Math Function1/1 -> Switch/1
  Demux1/2 -> Mux1/2
  Power/1 -> Switch1/1
  Power1/1 -> Switch1/3
  pump Swicht/1 -> Switch1/2
  feedback  flow rate/1 -> Demux2/1
  Demux2/2 -> Terminator4/1
  Demux1/1 -> Sum3/2
  Sum8/1 -> Sum4/2
  Sum4/1 -> Divide3/1
  Gain2/1 -> Sum2/1, Sum4/1, Sum7/1
  Demux2/1 -> Math Function5/1, Divide1/4
  Sum1/1 -> Divide/3
  Constant5/1 -> Divide/1
  Gain1/1 -> Sum1/2
  Math Function/1 -> Gain1/1
  Divide/1 -> Mux/1
  Math Function5/1 -> Product3/1
  Product3/1 -> Math Function7/1
  Constant3/1 -> Sum5/2
  Math Function7/1 -> Sum7/2
  Sum7/1 -> Divide1/3
  Sum5/1 -> Divide1/2
  Integrator/1 -> current1/1, Sum6/3
  Constant6/1 -> Sum6/1
  Averia helice obstruida/1 -> Switch2/2, Switch3/2
  [ON] -> Product1/2
  Product1/1 -> Switch2/3
  Constant7/1 -> Product1/1
  Power2/1 -> Switch3/3
  Abs/1 -> Divide1/1
  Switch3/1 -> Math Function2/1
  Divide1/1 -> Switch2/1
  Switch2/1 -> Mux/2
  Switch1/1 -> [ON]
  [ON] -> Divide/2
  Sum6/1 -> Gain3/1
  Gain3/1 -> Integrator/1
  Gain5/1 -> Sum6/2
  Math Function6/1 -> Gain5/1

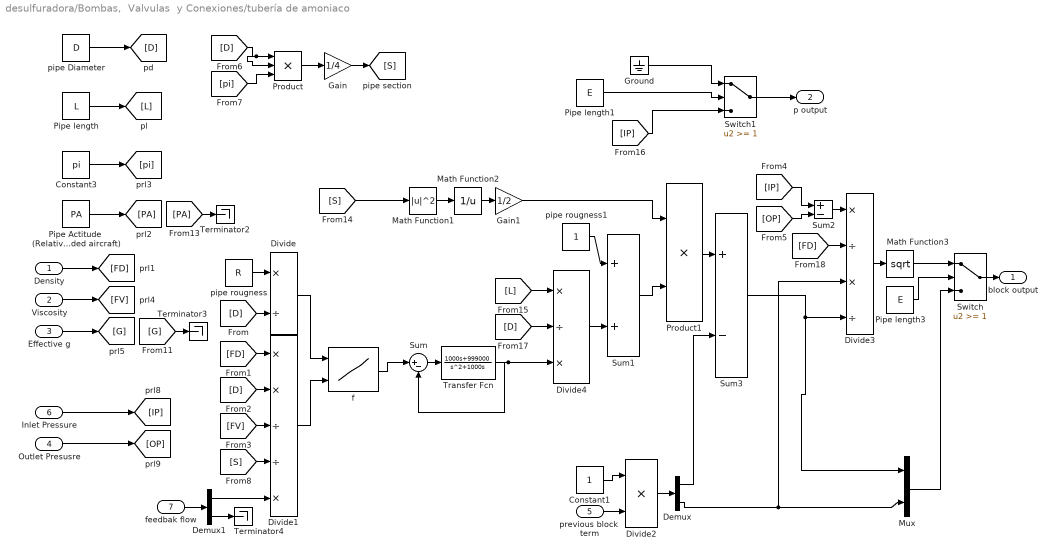
== system desulfuradora/Bombas,  Valvulas  y Conexiones/tubería de amoniaco ==
  Density : Inport
  Viscosity : Inport  Port=2
  Effective g : Inport  Port=3
  Outlet Presusre : Inport  Port=4
  previous block  term : Inport  Port=5
  Inlet Pressure : Inport  Port=6
  feedbak flow : Inport  Port=7
  Constant1 : Constant
  Constant3 : Constant  Value=pi
  Demux : Demux  Outputs=2
  Demux1 : Demux  Outputs=2
  Divide : Product  Inputs=*/
  Divide1 : Product  Inputs=**//*
  Divide2 : Product  Inputs=**
  Divide3 : Product  Inputs=*/*/
  Divide4 : Product  Inputs=*/*
  Gain : Gain  Gain=1/4
  Gain1 : Gain  Gain=1/2
  Ground : Ground
  Math Function1 : Math  Operator=magnitude^2  SaturateOnIntegerOverflow=on
  Math Function2 : Math  Operator=reciprocal  SaturateOnIntegerOverflow=on
  Math Function3 : Math  Operator=sqrt  SaturateOnIntegerOverflow=on
  Mux : Mux  Inputs=2
  Pipe Actitude  (Relative to landed aircraft) : Constant  Value=PA
  Pipe length : Constant  Value=L
  Pipe length1 : Constant  Value=E
  Pipe length3 : Constant  Value=E
  Product : Product  Inputs=3  RndMeth=Zero
  Product1 : Product  RndMeth=Zero
  Sum : Sum  Inputs=|+-
  Sum1 : Sum
  Sum2 : Sum  Inputs=+-
  Sum3 : Sum  Inputs=+-
  Switch : Switch  Threshold=1
  Switch1 : Switch  Threshold=1
  Terminator2 : Terminator
  Terminator3 : Terminator
  Terminator4 : Terminator
  Transfer Fcn : TransferFcn  Numerator=[1000 999000]  Denominator=[1 1000 0]
  f : Lookup2D  RowIndex=eps_d  ColumnIndex=re  Table=tabla
  pipe Diameter : Constant  Value=D
  pipe rougness : Constant  Value=R
  pipe rougness1 : Constant
  block output : Outport
  p output : Outport  Port=2
  wires:
  Divide/1 -> f/1
  Divide1/1 -> f/2
  pipe Diameter/1 -> [D]
  Constant3/1 -> [pi]
  Pipe length/1 -> [L]
  Pipe Actitude  (Relative to landed aircraft)/1 -> [PA]
  Density/1 -> [FD]
  Viscosity/1 -> [FV]
  Effective g/1 -> [G]
  Inlet Pressure/1 -> [IP]
  pipe rougness/1 -> Divide/1
  [D] -> Divide/2
  [FD] -> Divide1/1
  [D] -> Divide1/2
  [FV] -> Divide1/3
  [D] -> Product/1, Product/2
  Product/1 -> Gain/1
  Gain/1 -> [S]
  [S] -> Divide1/4
  [PA] -> Terminator2/1
  [L] -> Divide4/1
  [G] -> Terminator3/1
  [D] -> Divide4/2
  Outlet Presusre/1 -> [OP]
  [OP] -> Sum2/2
  [IP] -> Sum2/1
  Switch/1 -> block output/1
  Pipe length3/1 -> Switch/2
  Math Function1/1 -> Math Function2/1
  Math Function2/1 -> Gain1/1
  [S] -> Math Function1/1
  Gain1/1 -> Product1/1
  previous block  term/1 -> Divide2/2
  Constant1/1 -> Divide2/1
  Divide2/1 -> Demux/1
  Demux/2 -> Mux/2, Divide3/3
  Mux/1 -> Switch/3
  Divide4/1 -> Sum1/2
  pipe rougness1/1 -> Sum1/1
  Sum1/1 -> Product1/2
  Product1/1 -> Sum3/1
  Demux/1 -> Sum3/2
  Sum3/1 -> Divide3/4, Mux/1
  Sum2/1 -> Divide3/1
  [FD] -> Divide3/2
  Switch1/1 -> p output/1
  Pipe length1/1 -> Switch1/2
  Ground/1 -> Switch1/1
  [IP] -> Switch1/3
  [pi] -> Product/3
  Math Function3/1 -> Switch/1
  Divide3/1 -> Math Function3/1
  Transfer Fcn/1 -> Sum/2, Divide4/3
  Sum/1 -> Transfer Fcn/1
  f/1 -> Sum/1
  Demux1/1 -> Divide1/5
  feedbak flow/1 -> Demux1/1
  Demux1/2 -> Terminator4/1

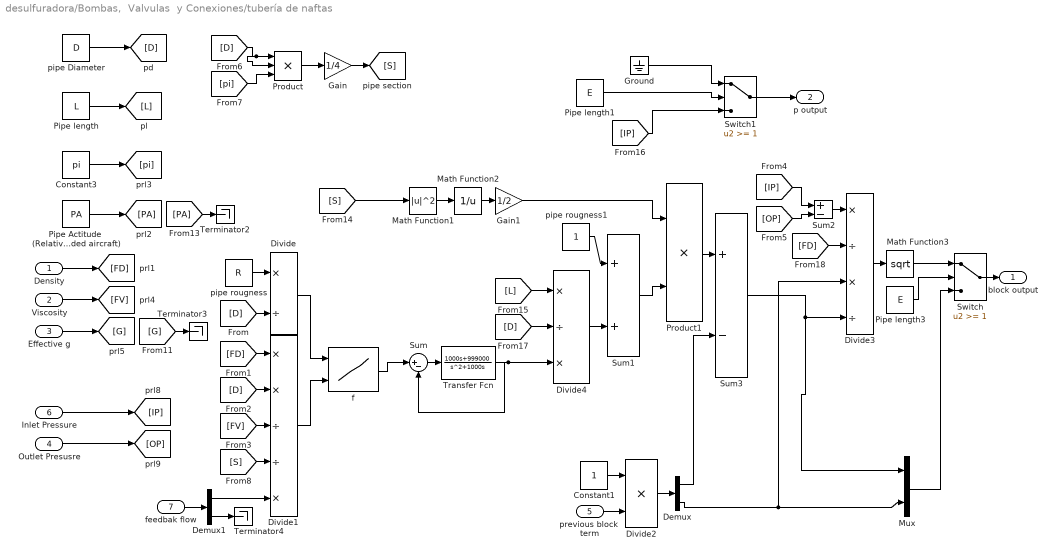
== system desulfuradora/Bombas,  Valvulas  y Conexiones/tubería de naftas ==
  Density : Inport
  Viscosity : Inport  Port=2
  Effective g : Inport  Port=3
  Outlet Presusre : Inport  Port=4
  previous block  term : Inport  Port=5
  Inlet Pressure : Inport  Port=6
  feedbak flow : Inport  Port=7
  Constant1 : Constant
  Constant3 : Constant  Value=pi
  Demux : Demux  Outputs=2
  Demux1 : Demux  Outputs=2
  Divide : Product  Inputs=*/
  Divide1 : Product  Inputs=**//*
  Divide2 : Product  Inputs=**
  Divide3 : Product  Inputs=*/*/
  Divide4 : Product  Inputs=*/*
  Gain : Gain  Gain=1/4
  Gain1 : Gain  Gain=1/2
  Ground : Ground
  Math Function1 : Math  Operator=magnitude^2  SaturateOnIntegerOverflow=on
  Math Function2 : Math  Operator=reciprocal  SaturateOnIntegerOverflow=on
  Math Function3 : Math  Operator=sqrt  SaturateOnIntegerOverflow=on
  Mux : Mux  Inputs=2
  Pipe Actitude  (Relative to landed aircraft) : Constant  Value=PA
  Pipe length : Constant  Value=L
  Pipe length1 : Constant  Value=E
  Pipe length3 : Constant  Value=E
  Product : Product  Inputs=3  RndMeth=Zero
  Product1 : Product  RndMeth=Zero
  Sum : Sum  Inputs=|+-
  Sum1 : Sum
  Sum2 : Sum  Inputs=+-
  Sum3 : Sum  Inputs=+-
  Switch : Switch  Threshold=1
  Switch1 : Switch  Threshold=1
  Terminator2 : Terminator
  Terminator3 : Terminator
  Terminator4 : Terminator
  Transfer Fcn : TransferFcn  Numerator=[1000 999000]  Denominator=[1 1000 0]
  f : Lookup2D  RowIndex=eps_d  ColumnIndex=re  Table=tabla
  pipe Diameter : Constant  Value=D
  pipe rougness : Constant  Value=R
  pipe rougness1 : Constant
  block output : Outport
  p output : Outport  Port=2
  wires:
  Divide/1 -> f/1
  Divide1/1 -> f/2
  pipe Diameter/1 -> [D]
  Constant3/1 -> [pi]
  Pipe length/1 -> [L]
  Pipe Actitude  (Relative to landed aircraft)/1 -> [PA]
  Density/1 -> [FD]
  Viscosity/1 -> [FV]
  Effective g/1 -> [G]
  Inlet Pressure/1 -> [IP]
  pipe rougness/1 -> Divide/1
  [D] -> Divide/2
  [FD] -> Divide1/1
  [D] -> Divide1/2
  [FV] -> Divide1/3
  [D] -> Product/1, Product/2
  Product/1 -> Gain/1
  Gain/1 -> [S]
  [S] -> Divide1/4
  [PA] -> Terminator2/1
  [L] -> Divide4/1
  [G] -> Terminator3/1
  [D] -> Divide4/2
  Outlet Presusre/1 -> [OP]
  [OP] -> Sum2/2
  [IP] -> Sum2/1
  Switch/1 -> block output/1
  Pipe length3/1 -> Switch/2
  Math Function1/1 -> Math Function2/1
  Math Function2/1 -> Gain1/1
  [S] -> Math Function1/1
  Gain1/1 -> Product1/1
  previous block  term/1 -> Divide2/2
  Constant1/1 -> Divide2/1
  Divide2/1 -> Demux/1
  Demux/2 -> Mux/2, Divide3/3
  Mux/1 -> Switch/3
  Divide4/1 -> Sum1/2
  pipe rougness1/1 -> Sum1/1
  Sum1/1 -> Product1/2
  Product1/1 -> Sum3/1
  Demux/1 -> Sum3/2
  Sum3/1 -> Divide3/4, Mux/1
  Sum2/1 -> Divide3/1
  [FD] -> Divide3/2
  Switch1/1 -> p output/1
  Pipe length1/1 -> Switch1/2
  Ground/1 -> Switch1/1
  [IP] -> Switch1/3
  [pi] -> Product/3
  Math Function3/1 -> Switch/1
  Divide3/1 -> Math Function3/1
  Transfer Fcn/1 -> Sum/2, Divide4/3
  Sum/1 -> Transfer Fcn/1
  f/1 -> Sum/1
  Demux1/1 -> Divide1/5
  feedbak flow/1 -> Demux1/1
  Demux1/2 -> Terminator4/1

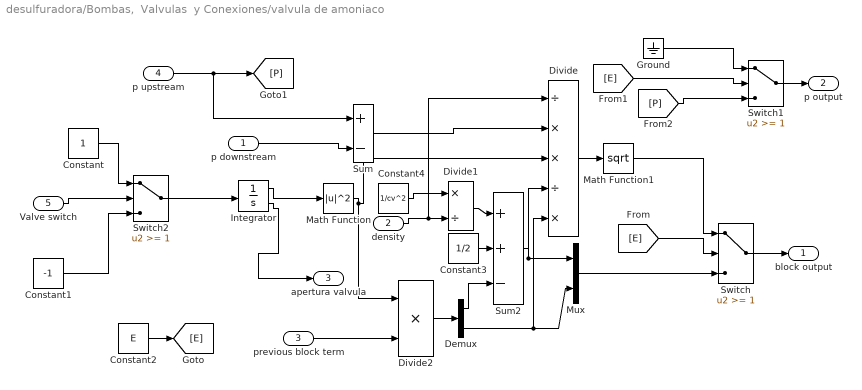
== system desulfuradora/Bombas,  Valvulas  y Conexiones/valvula de amoniaco ==
  p downstream : Inport
  " density" : Inport  Port=2
  previous block term : Inport  Port=3
  p upstream : Inport  Port=4
  Valve switch : Inport  Port=5
  Constant : Constant
  Constant1 : Constant  Value=-1
  Constant2 : Constant  Value=E
  Constant3 : Constant  Value=1/2
  Constant4 : Constant  Value=1/cv^2
  Demux : Demux  Outputs=2
  Divide : Product  Inputs=/**/*
  Divide1 : Product  Inputs=*/
  Divide2 : Product  Inputs=**
  Ground : Ground
  Integrator : Integrator  LimitOutput=on  UpperSaturationLimit=A  LowerSaturationLimit=0  ShowSaturationPort=on
  Math Function : Math  Operator=magnitude^2  SaturateOnIntegerOverflow=on
  Math Function1 : Math  Operator=sqrt  SaturateOnIntegerOverflow=on
  Mux : Mux  Inputs=2
  Sum : Sum  Inputs=+-
  Sum2 : Sum  Inputs=++-
  Switch : Switch  Threshold=1
  Switch1 : Switch  Threshold=1
  Switch2 : Switch  Threshold=1
  block output : Outport
  p output : Outport  Port=2
  apertura valvula : Outport  Port=3
  wires:
  Constant3/1 -> Sum2/2
  Sum2/1 -> Mux/1, Divide/4
  Math Function/1 -> Divide2/1, Divide/3
  Divide1/1 -> Sum2/1
  Constant4/1 -> Divide1/1
  " density"/1 -> Divide1/2, Divide/1
  Switch1/1 -> p output/1
  Constant2/1 -> [E]
  [E] -> Switch1/2
  Ground/1 -> Switch1/1
  p upstream/1 -> [P], Sum/1
  [P] -> Switch1/3
  Constant/1 -> Switch2/1
  Switch2/1 -> Integrator/1
  Constant1/1 -> Switch2/3
  Valve switch/1 -> Switch2/2
  p downstream/1 -> Sum/2
  [E] -> Switch/2
  previous block term/1 -> Divide2/2
  Divide2/1 -> Demux/1
  Demux/1 -> Sum2/3
  Demux/2 -> Mux/2, Divide/5
  Switch/1 -> block output/1
  Mux/1 -> Switch/3
  Sum/1 -> Divide/2
  Divide/1 -> Math Function1/1
  Math Function1/1 -> Switch/1
  Integrator/1 -> Math Function/1
  Integrator/2 -> apertura valvula/1

== system desulfuradora/Bombas,  Valvulas  y Conexiones/valvula de naftas ==
  p downstream : Inport
  " density" : Inport  Port=2
  prev. block term : Inport  Port=3
  p upstream : Inport  Port=4
  Valve switch : Inport  Port=5
  Constant : Constant
  Constant1 : Constant  Value=-1
  Constant2 : Constant  Value=E
  Constant3 : Constant  Value=1/2
  Constant4 : Constant  Value=1/cv^2
  Demux : Demux  Outputs=2
  Divide : Product  Inputs=/**/*
  Divide1 : Product  Inputs=*/
  Divide2 : Product  Inputs=**
  Ground : Ground
  Integrator : Integrator  LimitOutput=on  UpperSaturationLimit=A  LowerSaturationLimit=0  ShowSaturationPort=on
  Math Function : Math  Operator=magnitude^2  SaturateOnIntegerOverflow=on
  Math Function1 : Math  Operator=sqrt  SaturateOnIntegerOverflow=on
  Mux : Mux  Inputs=2
  Sum : Sum  Inputs=+-
  Sum2 : Sum  Inputs=++-
  Switch : Switch  Threshold=1
  Switch1 : Switch  Threshold=1
  Switch2 : Switch  Threshold=1
  block output : Outport
  p output : Outport  Port=2
  apertura valvula : Outport  Port=3
  wires:
  Constant3/1 -> Sum2/2
  Sum2/1 -> Mux/1, Divide/4
  Math Function/1 -> Divide2/1, Divide/3
  Divide1/1 -> Sum2/1
  Constant4/1 -> Divide1/1
  " density"/1 -> Divide1/2, Divide/1
  Switch1/1 -> p output/1
  Constant2/1 -> [E]
  [E] -> Switch1/2
  Ground/1 -> Switch1/1
  p upstream/1 -> [P], Sum/1
  [P] -> Switch1/3
  Constant/1 -> Switch2/1
  Valve switch/1 -> Switch2/2
  p downstream/1 -> Sum/2
  [E] -> Switch/2
  prev. block term/1 -> Divide2/2
  Divide2/1 -> Demux/1
  Demux/1 -> Sum2/3
  Demux/2 -> Mux/2, Divide/5
  Switch/1 -> block output/1
  Mux/1 -> Switch/3
  Sum/1 -> Divide/2
  Divide/1 -> Math Function1/1
  Math Function1/1 -> Switch/1
  Integrator/1 -> Math Function/1
  Switch2/1 -> Integrator/1
  Constant1/1 -> Switch2/3
  Integrator/2 -> apertura valvula/1
